simulink model "testbed_simulink_model"  (R2021a)
settings: Solver=FixedStepAuto  StartTime=0.0  StopTime=3  RelTol=1e-3
InitFcn:
  | fsw=10e3;
  | Ts=1/(fsw*50);
  | Vodref=220*sqrt(2);
  | Vdc=700;
  | w0=2*pi*50;
  | 
  | Lf=3.5e-3;
  | Rf=0.1;
  | Cf=50e-6;
  | Lc=0.35e-3;
  | Rc=0.05;
  | 
  | Tci=4/(2*pi*fsw);
  | wci=1/Tci;
  | Kpc=Lf*wci;
  | Kic=Rf*wci;
  | 
  | pm=50;
  | wcv=1/Tci*(1-sind(pm))/(1+sind(pm));
  | wgc=sqrt(wcv*wci);
  | Kpv=Cf*wgc;
  | Kiv=Kpv*wcv;
  | 
  | mp1=5e-5;
  | nq1=3e-3;
  | mp2=5e-5;
  | nq2=3e-3;
  | mp3=5e-5;
  | nq3=3e-3;
libraries: spsabctodq0Lib x15, pid_lib x12, spsThreePhaseSeriesRLCBranchLib x11, spsThreePhaseVIMeasurementLib x6, spsThreePhaseSeriesRLCLoadLib x5, spsThreePhaseBreakerLib x4, spsDCVoltageSourceLib x3, spsGroundLib x3, spsPWMGenerator2LevelLib x3, spsUniversalBridgeLib x3, spsdq0toabcLib x3, spsThreePhaseFaultLib x1
(part 1 of 2)
settings Model: SimulationMode=accelerator  Creator=HP omen  LastModifiedBy=chigo
settings SolverCC: AlgebraicLoopSolver=TrustRegion
settings DataIOCC: ReturnWorkspaceOutputs=off

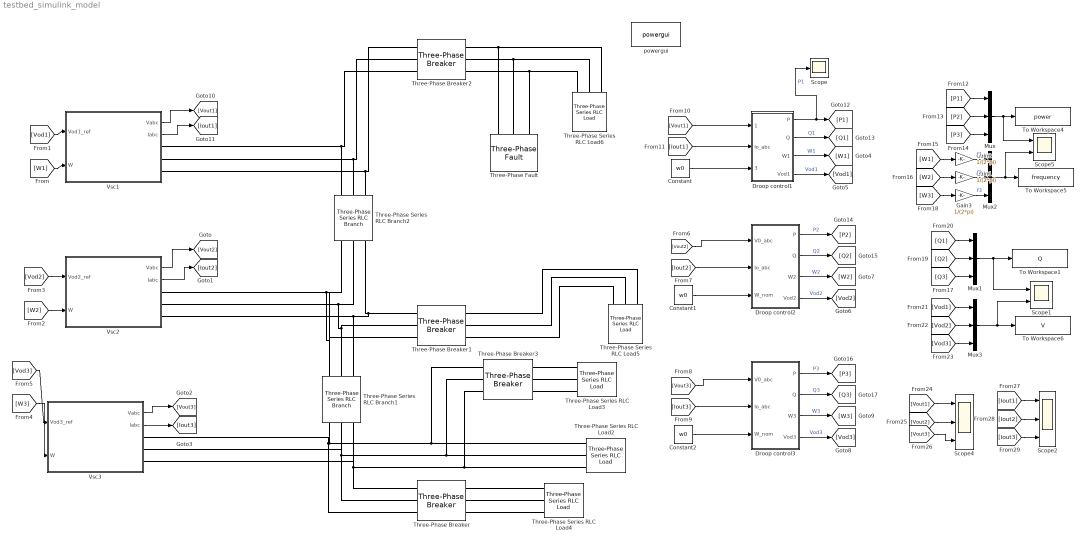
== system testbed_simulink_model ==
  Constant : Constant  Value=w0
  Constant1 : Constant  Value=w0
  Constant2 : Constant  Value=w0
  Droop control1 : Subsystem
  Droop control2 : Subsystem
  Droop control3 : Subsystem
  Gain1 : Gain  Gain=1/(2*pi)
  Gain2 : Gain  Gain=1/(2*pi)
  Gain3 : Gain  Gain=1/(2*pi)
  Mux{,1..3} (4 alike) : Mux  Inputs=3
  Scope : Scope
  Scope1 : Scope  NumInputPorts=2
  Scope2 : Scope  NumInputPorts=3
  Scope4 : Scope  NumInputPorts=3
  Scope5 : Scope  NumInputPorts=2
  Three-Phase Series RLC Branch1 : spsThreePhaseSeriesRLCBranchLib/Three-Phase Series RLC Branch  LConnTagsString=A|B|C  RConnTagsString=A|B|C  BranchType=RL  Resistance=0.15  Inductance=3.5e-4  Capacitance=1e-6  Measurements=Branch voltages
  Three-Phase Series RLC Branch2 : spsThreePhaseSeriesRLCBranchLib/Three-Phase Series RLC Branch  LConnTagsString=A|B|C  RConnTagsString=A|B|C  BranchType=RL  Resistance=0.15  Inductance=3.5e-4  Capacitance=1e-6  Measurements=None
  Three-Phase Series RLC Load2 : spsThreePhaseSeriesRLCLoadLib/Three-Phase Series RLC Load  LConnTagsString=A|B|C  Configuration=Y (grounded)  NominalVoltage=380  Vabc=[1e3 1e3 1e3]  Vabcp=[1e3 1e3 1e3]  NominalFrequency=50  UnbalancedPower=off  ActivePower=6.3e3  InductivePower=1e3  CapacitivePower=0  Pabc=[10e3 9e3 11e3]  QLabc=[100 90 110]  QCabc=[100 90 110]  Pabcp=[10e3 9e3 11e3]  QLabcp=[100 90 110]  QCabcp=[100 90 110]  Measurements=None  LoadType=constant Z
  Three-Phase Series RLC Load3 : spsThreePhaseSeriesRLCLoadLib/Three-Phase Series RLC Load  LConnTagsString=A|B|C  Configuration=Y (grounded)  NominalVoltage=380  Vabc=[1e3 1e3 1e3]  Vabcp=[1e3 1e3 1e3]  NominalFrequency=50  UnbalancedPower=off  ActivePower=2.3e3  InductivePower=0.3e3  CapacitivePower=0  Pabc=[10e3 9e3 11e3]  QLabc=[100 90 110]  QCabc=[100 90 110]  Pabcp=[10e3 9e3 11e3]  QLabcp=[100 90 110]  QCabcp=[100 90 110]  Measurements=None  LoadType=constant Z
  Three-Phase Series RLC Load4 : spsThreePhaseSeriesRLCLoadLib/Three-Phase Series RLC Load  LConnTagsString=A|B|C  Configuration=Y (grounded)  NominalVoltage=380  Vabc=[1e3 1e3 1e3]  Vabcp=[1e3 1e3 1e3]  NominalFrequency=50  UnbalancedPower=off  ActivePower=5.8e3  InductivePower=0.2e3  CapacitivePower=0  Pabc=[10e3 9e3 11e3]  QLabc=[100 90 110]  QCabc=[100 90 110]  Pabcp=[10e3 9e3 11e3]  QLabcp=[100 90 110]  QCabcp=[100 90 110]  Measurements=None  LoadType=constant Z
  Three-Phase Series RLC Load5 : spsThreePhaseSeriesRLCLoadLib/Three-Phase Series RLC Load  LConnTagsString=A|B|C  Configuration=Y (grounded)  NominalVoltage=380  Vabc=[1e3 1e3 1e3]  Vabcp=[1e3 1e3 1e3]  NominalFrequency=50  UnbalancedPower=off  ActivePower=5.8e3  InductivePower=0.2e3  CapacitivePower=0  Pabc=[10e3 9e3 11e3]  QLabc=[100 90 110]  QCabc=[100 90 110]  Pabcp=[10e3 9e3 11e3]  QLabcp=[100 90 110]  QCabcp=[100 90 110]  Measurements=None  LoadType=constant Z
  Three-Phase Series RLC Load6 : spsThreePhaseSeriesRLCLoadLib/Three-Phase Series RLC Load  LConnTagsString=A|B|C  Configuration=Y (grounded)  NominalVoltage=380  Vabc=[1e3 1e3 1e3]  Vabcp=[1e3 1e3 1e3]  NominalFrequency=50  UnbalancedPower=off  ActivePower=5.8e3  InductivePower=0.2e3  CapacitivePower=0  Pabc=[10e3 9e3 11e3]  QLabc=[100 90 110]  QCabc=[100 90 110]  Pabcp=[10e3 9e3 11e3]  QLabcp=[100 90 110]  QCabcp=[100 90 110]  Measurements=None  LoadType=constant Z
  Three-Phase Breaker : spsThreePhaseBreakerLib/Three-Phase Breaker  InitialState=open  SwitchA=on  SwitchB=on  SwitchC=on  SwitchTimes=0  External=off  BreakerResistance=0.01  SnubberResistance=1e6  SnubberCapacitance=inf  Measurements=None
  Three-Phase Breaker1 : spsThreePhaseBreakerLib/Three-Phase Breaker  InitialState=open  SwitchA=on  SwitchB=on  SwitchC=on  SwitchTimes=0  External=off  BreakerResistance=0.01  SnubberResistance=1e6  SnubberCapacitance=inf  Measurements=None
  Three-Phase Breaker2 : spsThreePhaseBreakerLib/Three-Phase Breaker  InitialState=closed  SwitchA=on  SwitchB=on  SwitchC=on  SwitchTimes=0  External=off  BreakerResistance=0.01  SnubberResistance=1e6  SnubberCapacitance=inf  Measurements=None
  Three-Phase Breaker3 : spsThreePhaseBreakerLib/Three-Phase Breaker  InitialState=closed  SwitchA=on  SwitchB=on  SwitchC=on  SwitchTimes=0  External=off  BreakerResistance=0.01  SnubberResistance=1e6  SnubberCapacitance=inf  Measurements=None
  Three-Phase Fault : spsThreePhaseFaultLib/Three-Phase Fault  InitialStates=0  FaultA=off  FaultB=off  FaultC=off  GroundFault=off  SwitchTimes=[2]  External=off  SwitchStatus=NaN  FaultResistance=0.001  GroundResistance=0.01  SnubberResistance=1e6  SnubberCapacitance=inf  Measurements=None
  To Workspace1 : ToWorkspace  VariableName=Q  SaveFormat=Structure With Time  SampleTime=-1
  To Workspace4 : ToWorkspace  VariableName=power  SaveFormat=Structure With Time  SampleTime=-1
  To Workspace5 : ToWorkspace  VariableName=frequency  SaveFormat=Structure With Time  SampleTime=-1
  To Workspace6 : ToWorkspace  VariableName=V  SaveFormat=Structure With Time  SampleTime=-1
  Vsc1 : Subsystem
  Vsc2 : Subsystem
  Vsc3 : Subsystem
  powergui : spspowerguiLib/powergui  Priority=1  SimulationMode=Discrete  SampleTime=Ts  frequency=60  Iterations=50  frequencyindice=0  Pbase=100e6  ErrMax=1e-4  UnitsV=kV  UnitsW=MW  buscounter=0  FunctionMessages=off  echomessages=off  EnableUseOfTLC=off  CurrentSourceSwitches=off  DisableSnubberDevices=off  DisableRonSwitches=off  DisableVfSwitches=off  DisplayEquations=off  AutomaticDiscreteSolvers=off  SolverType=Tustin/Backward Euler (TBE)  Interpol=off  ExternalGateDelay=off  methode=off  Ts=100  x0status=blocks  SPID=on  SwTol=0  HookPort=off  NonlinearTolerance=1e-4  nMaxIteration=100  ContinueOnMaxIteration=off  RestoreLinks=warning  ResistiveCurrentMeasurement=off  Frange=[0:2:500]  Ylog=off  Xlog=on  ShowGrid=off  save=off  variable=ZData  structure=0  ZoomFFT=off  StartTime=0.0  cycles=1  DisplayStyle=1  fundamental=60  FreqAxis=off  MaxFrequency=1000  frequencyindicesteady=1  RmsSteady=1  display=off
  wires:
  Vsc2/1(Vabc) -> [Vout2]
  Vsc3/1(Vabc) -> [Vout3]
  Vsc2/2(Iabc) -> [Iout2]
  Vsc3/2(Iabc) -> [Iout3]
  Constant/1 -> Droop control1/3(W_nom)
  Droop control1/3(W1) -> [W1]  "W1"
  Droop control1/4(Vod1) -> [Vod1]  "Vod1"
  [Vod1] -> Vsc1/1(Vod1_ref)
  [W1] -> Vsc1/2(W)
  [W3] -> Vsc3/2(W)
  [Vod3] -> Vsc3/1(Vod3_ref)
  [W2] -> Vsc2/2(W)
  [Vod2] -> Vsc2/1(Vod2_ref)
  [Vout3] -> Droop control3/1(V0_abc)
  [Iout3] -> Droop control3/2(Io_abc)
  [Vout2] -> Droop control2/1(V0_abc)
  [Iout2] -> Droop control2/2(Io_abc)
  Constant1/1 -> Droop control2/3(W_nom)
  Constant2/1 -> Droop control3/3(W_nom)
  Droop control2/3(W2) -> [W2]  "W2"
  Droop control2/4(Vod2) -> [Vod2]  "Vod2"
  Droop control3/4(Vod3) -> [Vod3]  "Vod3"
  Droop control3/3(W3) -> [W3]  "W3"
  Vsc1/1(Vabc) -> [Vout1]
  Vsc1/2(Iabc) -> [Iout1]
  [Iout1] -> Droop control1/2(Io_abc)
  [Vout1] -> Droop control1/1(V0_abc)
  Droop control1/1(P) -> Scope/1, [P1]  "P1"
  Droop control1/2(Q) -> [Q1]  "Q1"
  Droop control2/1(P) -> [P2]  "P2"
  Droop control2/2(Q) -> [Q2]  "Q2"
  Droop control3/1(P) -> [P3]  "P3"
  Droop control3/2(Q) -> [Q3]  "Q3"
  [W1] -> Gain2/1
  [W2] -> Gain1/1
  [W3] -> Gain3/1
  [P2] -> Mux/2
  [P1] -> Mux/1
  [P3] -> Mux/3
  [Q1] -> Mux1/1
  [Q2] -> Mux1/2
  [Q3] -> Mux1/3
  Gain2/1 -> Mux2/1  "f1"
  Gain1/1 -> Mux2/2  "f2"
  Gain3/1 -> Mux2/3  "f3"
  [Vod1] -> Mux3/1
  [Vod2] -> Mux3/2
  [Vod3] -> Mux3/3
  Mux1/1 -> To Workspace1/1, Scope1/1
  Mux3/1 -> To Workspace6/1, Scope1/2
  Mux/1 -> Scope5/1, To Workspace4/1
  Mux2/1 -> To Workspace5/1, Scope5/2
  [Vout1] -> Scope4/1
  [Vout2] -> Scope4/2
  [Vout3] -> Scope4/3
  [Iout1] -> Scope2/1
  [Iout2] -> Scope2/2
  [Iout3] -> Scope2/3
  connections:
  Three-Phase Breaker2/LConn1 -- Vsc1/RConn1 -- Three-Phase Series RLC Branch2/LConn1
  Three-Phase Series RLC Load2/LConn1 -- Three-Phase Breaker3/LConn1 -- Vsc3/RConn1 -- Three-Phase Breaker/LConn1 -- Three-Phase Series RLC Branch1/RConn1
  Three-Phase Series RLC Branch2/LConn2 -- Three-Phase Breaker2/LConn2 -- Vsc1/RConn2
  Three-Phase Series RLC Branch2/LConn3 -- Three-Phase Breaker2/LConn3 -- Vsc1/RConn3
  Three-Phase Series RLC Load2/LConn2 -- Three-Phase Breaker3/LConn2 -- Three-Phase Series RLC Branch1/RConn2 -- Vsc3/RConn2 -- Three-Phase Breaker/LConn2
  Three-Phase Breaker/RConn3 -- Three-Phase Series RLC Load4/LConn1
  Three-Phase Breaker/RConn2 -- Three-Phase Series RLC Load4/LConn2
  Three-Phase Breaker/RConn1 -- Three-Phase Series RLC Load4/LConn3
  Three-Phase Series RLC Load5/LConn1 -- Three-Phase Breaker1/RConn1
  Three-Phase Series RLC Load5/LConn2 -- Three-Phase Breaker1/RConn2
  Three-Phase Series RLC Load5/LConn3 -- Three-Phase Breaker1/RConn3
  Three-Phase Series RLC Load6/LConn1 -- Three-Phase Fault/LConn1 -- Three-Phase Breaker2/RConn1
  Three-Phase Series RLC Load6/LConn2 -- Three-Phase Breaker2/RConn2 -- Three-Phase Fault/LConn2
  Three-Phase Series RLC Load6/LConn3 -- Three-Phase Fault/LConn3 -- Three-Phase Breaker2/RConn3
  Three-Phase Series RLC Branch2/RConn3 -- Three-Phase Breaker1/LConn3 -- Vsc2/RConn3 -- Three-Phase Series RLC Branch1/LConn3
  Three-Phase Series RLC Branch2/RConn1 -- Vsc2/RConn1 -- Three-Phase Breaker1/LConn1 -- Three-Phase Series RLC Branch1/LConn1
  Three-Phase Series RLC Branch1/LConn2 -- Three-Phase Breaker1/LConn2 -- Vsc2/RConn2 -- Three-Phase Series RLC Branch2/RConn2
  Three-Phase Series RLC Load2/LConn3 -- Three-Phase Breaker3/LConn3 -- Three-Phase Series RLC Branch1/RConn3 -- Vsc3/RConn3 -- Three-Phase Breaker/LConn3
  Three-Phase Breaker3/RConn1 -- Three-Phase Series RLC Load3/LConn1
  Three-Phase Breaker3/RConn2 -- Three-Phase Series RLC Load3/LConn2
  Three-Phase Breaker3/RConn3 -- Three-Phase Series RLC Load3/LConn3

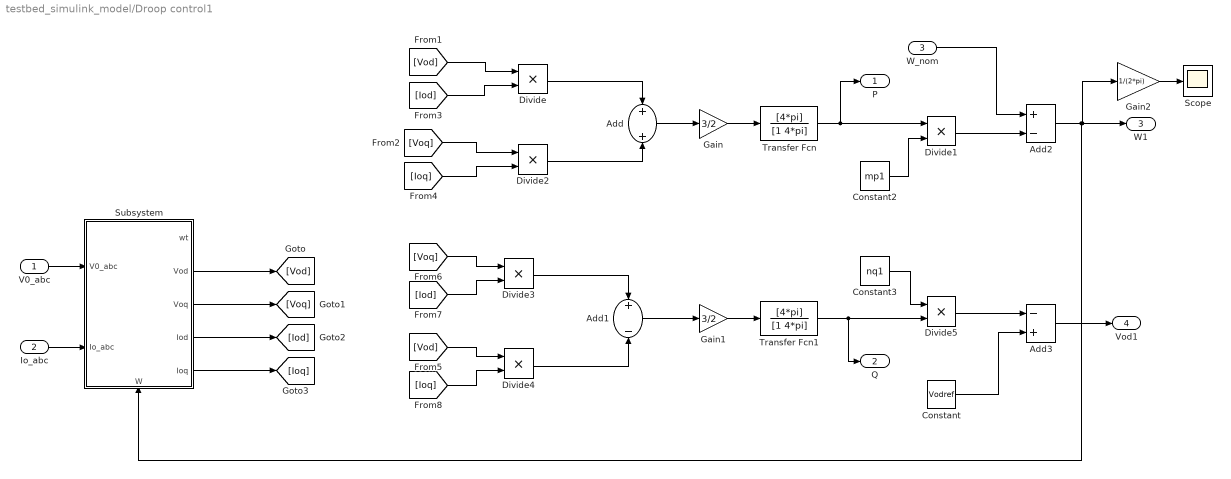
== system testbed_simulink_model/Droop control1 ==
  V0_abc : Inport
  Io_abc : Inport  Port=2
  W_nom : Inport  Port=3
  Add : Sum
  Add1 : Sum  Inputs=+-
  Add2 : Sum  Inputs=+-
  Add3 : Sum  Inputs=-+
  Constant : Constant  Value=Vodref
  Constant2 : Constant  Value=mp1
  Constant3 : Constant  Value=nq1
  Divide{,1..5} (6 alike) : Product  Inputs=**
  Gain : Gain  Gain=3/2
  Gain1 : Gain  Gain=3/2
  Gain2 : Gain  Gain=1/(2*pi)
  Scope : Scope
  Subsystem : Subsystem
      settings: PortSchema="{\"entries\":[{\"content\":{\"sides\":[{\"content\":{\"connectorIds\":[\"In1\",\"In2\"]},\"type\":\"ConnectorPlacement.EquallySpacedRectSide\",\"uuid\":\"3c0ce44c-1409-4df9-aab1-2e1a82b43481\"},{\"content\":{\"connectorIds\":[\"Out1\",\"Out2\",\"Out3\",\"Out4\",\"Out5\"],\"side\":\"RIGHT\"},\"type\":\"ConnectorPlacement.EquallySpacedRectSide\",\"uuid\":\"4a9336a4-679f-4f93-987c-a9f8549bd21c\"},{\"content\":{\"connectorIds\":[],\"side\":\"TOP\"},\"type\":\"ConnectorPlacement.EquallySpacedRectSide\",\"uuid\":\"6340f487-ff74-466e-845e-7d1050881641\"},{\"content\":{\"connectorIds\":[\"In3\"],\"side\":\"BOTTOM\"},\"type\":\"ConnectorPlacement.EquallySpacedRectSide\",\"uuid\":\"1e1d92d0-8955-434a-9fbd-76af504505ea\"}]},\"type\":\"ConnectorPlacement.EquallySpacedConnector\",\"uuid\":\"bfddd833-a64a-4f18-a4bd-88042aac52a3\"}],\"packageUris\":[\"http://schema.mathworks.com/mf0/Connector/R2020b\"],\"version\":\"1.0\"}"
  Transfer Fcn : TransferFcn  Numerator=[4*pi]  Denominator=[1 4*pi]
  Transfer Fcn1 : TransferFcn  Numerator=[4*pi]  Denominator=[1 4*pi]
  P : Outport
  Q : Outport  Port=2
  W1 : Outport  Port=3
  Vod1 : Outport  Port=4
  wires:
  Subsystem/2(Vod) -> [Vod]
  Subsystem/3(Voq) -> [Voq]
  Subsystem/4(Iod) -> [Iod]
  Subsystem/5(Ioq) -> [Ioq]
  [Vod] -> Divide/1
  [Iod] -> Divide/2
  [Voq] -> Divide2/1
  [Ioq] -> Divide2/2
  Divide/1 -> Add/1
  Divide2/1 -> Add/2
  Add/1 -> Gain/1
  [Voq] -> Divide3/1
  [Iod] -> Divide3/2
  [Vod] -> Divide4/1
  [Ioq] -> Divide4/2
  Divide3/1 -> Add1/1
  Divide4/1 -> Add1/2
  Add1/1 -> Gain1/1
  W_nom/1 -> Add2/1
  Divide1/1 -> Add2/2
  Divide5/1 -> Add3/1
  Constant/1 -> Add3/2
  Constant2/1 -> Divide1/2
  Constant3/1 -> Divide5/1
  Add2/1 -> Gain2/1, W1/1, Subsystem/3(W)
  Add3/1 -> Vod1/1
  Gain/1 -> Transfer Fcn/1
  Transfer Fcn/1 -> P/1, Divide1/1
  Gain1/1 -> Transfer Fcn1/1
  Transfer Fcn1/1 -> Q/1, Divide5/2
  Io_abc/1 -> Subsystem/2(Io_abc)
  V0_abc/1 -> Subsystem/1(V0_abc)
  Gain2/1 -> Scope/1

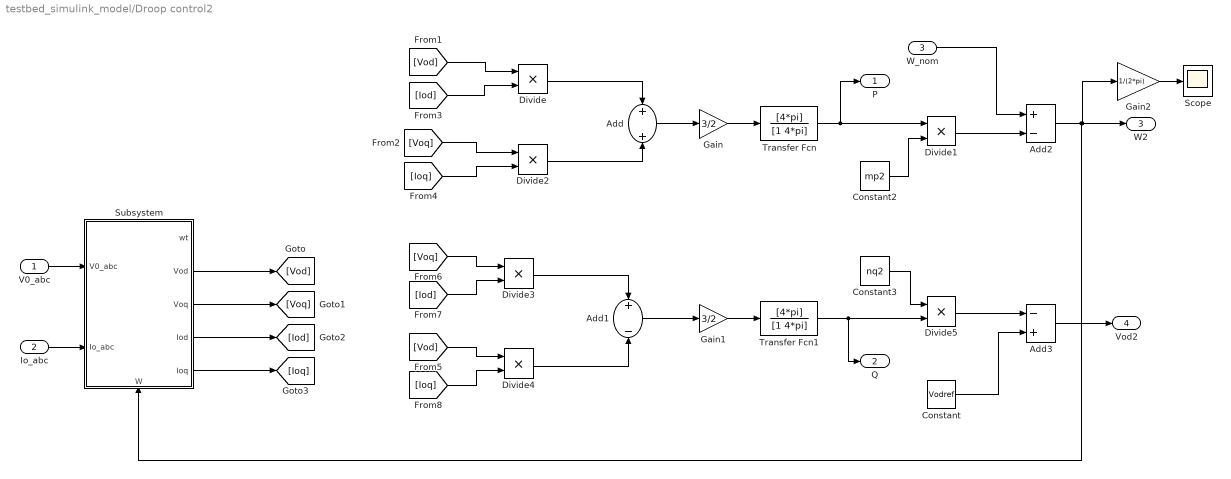
== system testbed_simulink_model/Droop control2 ==
  V0_abc : Inport
  Io_abc : Inport  Port=2
  W_nom : Inport  Port=3
  Add : Sum
  Add1 : Sum  Inputs=+-
  Add2 : Sum  Inputs=+-
  Add3 : Sum  Inputs=-+
  Constant : Constant  Value=Vodref
  Constant2 : Constant  Value=mp2
  Constant3 : Constant  Value=nq2
  Divide{,1..5} (6 alike) : Product  Inputs=**
  Gain : Gain  Gain=3/2
  Gain1 : Gain  Gain=3/2
  Gain2 : Gain  Gain=1/(2*pi)
  Scope : Scope
  Subsystem : Subsystem
      settings: PortSchema="{\"entries\":[{\"content\":{\"sides\":[{\"content\":{\"connectorIds\":[\"In1\",\"In2\"]},\"type\":\"ConnectorPlacement.EquallySpacedRectSide\",\"uuid\":\"3c0ce44c-1409-4df9-aab1-2e1a82b43481\"},{\"content\":{\"connectorIds\":[\"Out1\",\"Out2\",\"Out3\",\"Out4\",\"Out5\"],\"side\":\"RIGHT\"},\"type\":\"ConnectorPlacement.EquallySpacedRectSide\",\"uuid\":\"4a9336a4-679f-4f93-987c-a9f8549bd21c\"},{\"content\":{\"connectorIds\":[],\"side\":\"TOP\"},\"type\":\"ConnectorPlacement.EquallySpacedRectSide\",\"uuid\":\"6340f487-ff74-466e-845e-7d1050881641\"},{\"content\":{\"connectorIds\":[\"In3\"],\"side\":\"BOTTOM\"},\"type\":\"ConnectorPlacement.EquallySpacedRectSide\",\"uuid\":\"1e1d92d0-8955-434a-9fbd-76af504505ea\"}]},\"type\":\"ConnectorPlacement.EquallySpacedConnector\",\"uuid\":\"bfddd833-a64a-4f18-a4bd-88042aac52a3\"}],\"packageUris\":[\"http://schema.mathworks.com/mf0/Connector/R2020b\"],\"version\":\"1.0\"}"
  Transfer Fcn : TransferFcn  Numerator=[4*pi]  Denominator=[1 4*pi]
  Transfer Fcn1 : TransferFcn  Numerator=[4*pi]  Denominator=[1 4*pi]
  P : Outport
  Q : Outport  Port=2
  W2 : Outport  Port=3
  Vod2 : Outport  Port=4
  wires:
  Subsystem/2(Vod) -> [Vod]
  Subsystem/3(Voq) -> [Voq]
  Subsystem/4(Iod) -> [Iod]
  Subsystem/5(Ioq) -> [Ioq]
  [Vod] -> Divide/1
  [Iod] -> Divide/2
  [Voq] -> Divide2/1
  [Ioq] -> Divide2/2
  Divide/1 -> Add/1
  Divide2/1 -> Add/2
  Add/1 -> Gain/1
  [Voq] -> Divide3/1
  [Iod] -> Divide3/2
  [Vod] -> Divide4/1
  [Ioq] -> Divide4/2
  Divide3/1 -> Add1/1
  Divide4/1 -> Add1/2
  Add1/1 -> Gain1/1
  W_nom/1 -> Add2/1
  Divide1/1 -> Add2/2
  Divide5/1 -> Add3/1
  Constant/1 -> Add3/2
  Constant2/1 -> Divide1/2
  Constant3/1 -> Divide5/1
  Add2/1 -> Gain2/1, W2/1, Subsystem/3(W)
  Add3/1 -> Vod2/1
  Gain/1 -> Transfer Fcn/1
  Transfer Fcn/1 -> P/1, Divide1/1
  Gain1/1 -> Transfer Fcn1/1
  Transfer Fcn1/1 -> Q/1, Divide5/2
  Io_abc/1 -> Subsystem/2(Io_abc)
  V0_abc/1 -> Subsystem/1(V0_abc)
  Gain2/1 -> Scope/1

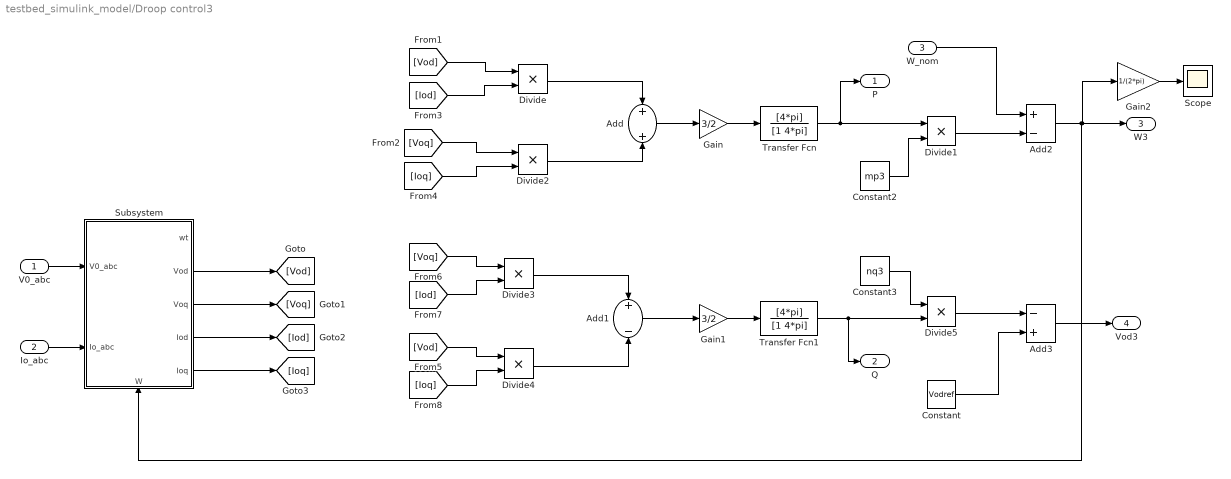
== system testbed_simulink_model/Droop control3 ==
  V0_abc : Inport
  Io_abc : Inport  Port=2
  W_nom : Inport  Port=3
  Add : Sum
  Add1 : Sum  Inputs=+-
  Add2 : Sum  Inputs=+-
  Add3 : Sum  Inputs=-+
  Constant : Constant  Value=Vodref
  Constant2 : Constant  Value=mp3
  Constant3 : Constant  Value=nq3
  Divide{,1..5} (6 alike) : Product  Inputs=**
  Gain : Gain  Gain=3/2
  Gain1 : Gain  Gain=3/2
  Gain2 : Gain  Gain=1/(2*pi)
  Scope : Scope
  Subsystem : Subsystem
      settings: PortSchema="{\"entries\":[{\"content\":{\"sides\":[{\"content\":{\"connectorIds\":[\"In1\",\"In2\"]},\"type\":\"ConnectorPlacement.EquallySpacedRectSide\",\"uuid\":\"3c0ce44c-1409-4df9-aab1-2e1a82b43481\"},{\"content\":{\"connectorIds\":[\"Out1\",\"Out2\",\"Out3\",\"Out4\",\"Out5\"],\"side\":\"RIGHT\"},\"type\":\"ConnectorPlacement.EquallySpacedRectSide\",\"uuid\":\"4a9336a4-679f-4f93-987c-a9f8549bd21c\"},{\"content\":{\"connectorIds\":[],\"side\":\"TOP\"},\"type\":\"ConnectorPlacement.EquallySpacedRectSide\",\"uuid\":\"6340f487-ff74-466e-845e-7d1050881641\"},{\"content\":{\"connectorIds\":[\"In3\"],\"side\":\"BOTTOM\"},\"type\":\"ConnectorPlacement.EquallySpacedRectSide\",\"uuid\":\"1e1d92d0-8955-434a-9fbd-76af504505ea\"}]},\"type\":\"ConnectorPlacement.EquallySpacedConnector\",\"uuid\":\"bfddd833-a64a-4f18-a4bd-88042aac52a3\"}],\"packageUris\":[\"http://schema.mathworks.com/mf0/Connector/R2020b\"],\"version\":\"1.0\"}"
  Transfer Fcn : TransferFcn  Numerator=[4*pi]  Denominator=[1 4*pi]
  Transfer Fcn1 : TransferFcn  Numerator=[4*pi]  Denominator=[1 4*pi]
  P : Outport
  Q : Outport  Port=2
  W3 : Outport  Port=3
  Vod3 : Outport  Port=4
  wires:
  Subsystem/2(Vod) -> [Vod]
  Subsystem/3(Voq) -> [Voq]
  Subsystem/4(Iod) -> [Iod]
  Subsystem/5(Ioq) -> [Ioq]
  [Vod] -> Divide/1
  [Iod] -> Divide/2
  [Voq] -> Divide2/1
  [Ioq] -> Divide2/2
  Divide/1 -> Add/1
  Divide2/1 -> Add/2
  Add/1 -> Gain/1
  [Voq] -> Divide3/1
  [Iod] -> Divide3/2
  [Vod] -> Divide4/1
  [Ioq] -> Divide4/2
  Divide3/1 -> Add1/1
  Divide4/1 -> Add1/2
  Add1/1 -> Gain1/1
  W_nom/1 -> Add2/1
  Divide1/1 -> Add2/2
  Divide5/1 -> Add3/1
  Constant/1 -> Add3/2
  Constant2/1 -> Divide1/2
  Constant3/1 -> Divide5/1
  Add2/1 -> Gain2/1, W3/1, Subsystem/3(W)
  Add3/1 -> Vod3/1
  Gain/1 -> Transfer Fcn/1
  Transfer Fcn/1 -> P/1, Divide1/1
  Gain1/1 -> Transfer Fcn1/1
  Transfer Fcn1/1 -> Q/1, Divide5/2
  Io_abc/1 -> Subsystem/2(Io_abc)
  V0_abc/1 -> Subsystem/1(V0_abc)
  Gain2/1 -> Scope/1

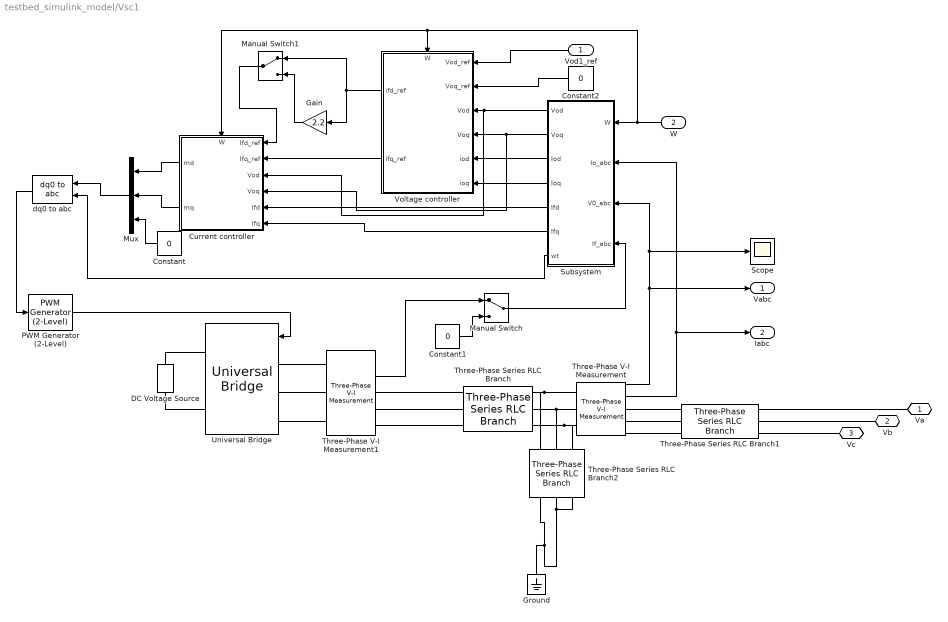
== system testbed_simulink_model/Vsc1 ==
  Vod1_ref : Inport
  W : Inport  Port=2
  Constant : Constant  Value=0
  Constant1 : Constant  Value=0
  Constant2 : Constant  Value=0
  Current controller : Subsystem
      settings: PortSchema="{\"entries\":[{\"content\":{\"sides\":[{\"content\":{\"connectorIds\":[\"In1\",\"In2\",\"In3\",\"In4\",\"In5\",\"In6\"]},\"type\":\"ConnectorPlacement.EquallySpacedRectSide\",\"uuid\":\"afbd0cd8-be12-4bd7-a6dd-f7dac5cf4512\"},{\"content\":{\"connectorIds\":[\"Out1\",\"Out2\"],\"side\":\"RIGHT\"},\"type\":\"ConnectorPlacement.EquallySpacedRectSide\",\"uuid\":\"a2288591-3041-41c1-b291-e9e060e5938f\"},{\"content\":{\"connectorIds\":[\"In7\"],\"side\":\"TOP\"},\"type\":\"ConnectorPlacement.EquallySpacedRectSide\",\"uuid\":\"6bd258a4-7022-4004-b2e3-8400b1f87dc6\"}]},\"type\":\"ConnectorPlacement.EquallySpacedConnector\",\"uuid\":\"ef76f81b-f821-49f2-9550-8127a934c8c3\"}],\"packageUris\":[\"http://schema.mathworks.com/mf0/Connector/R2020b\"],\"version\":\"1.0\"}"
  DC Voltage Source : spsDCVoltageSourceLib/DC Voltage Source  Amplitude=Vdc  Measurements=None
  Gain : Gain  Gain=2.2
  Ground : spsGroundLib/Ground  LConnTagsString=a
  Manual Switch : ManualSwitch
  Manual Switch1 : ManualSwitch
  Mux : Mux  Inputs=3
  PWM Generator (2-Level) : spsPWMGenerator2LevelLib/PWM Generator (2-Level)  ModulatorType=Three-phase bridge (6 pulses)  ModulatorMode=Unsynchronized  Fc=fsw  Pc=0  nF=27  MinMax="[ -1  1 ]"  SamplingTechnique=Natural  ModulatingSignals=off  m=0.8  Freq=60  Phase=0  Ts=0  ShowCarrierOutport=off
  Scope : Scope
  Subsystem : Subsystem
  Three-Phase Series RLC Branch : spsThreePhaseSeriesRLCBranchLib/Three-Phase Series RLC Branch  LConnTagsString=A|B|C  RConnTagsString=A|B|C  BranchType=RL  Resistance=Rf  Inductance=Lf  Capacitance=1e-6  Measurements=None
  Three-Phase Series RLC Branch1 : spsThreePhaseSeriesRLCBranchLib/Three-Phase Series RLC Branch  LConnTagsString=A|B|C  RConnTagsString=A|B|C  BranchType=RL  Resistance=Rc  Inductance=Lc  Capacitance=1e-6  Measurements=None
  Three-Phase Series RLC Branch2 : spsThreePhaseSeriesRLCBranchLib/Three-Phase Series RLC Branch  LConnTagsString=A|B|C  RConnTagsString=A|B|C  BranchType=C  Resistance=1  Inductance=1e-3  Capacitance=Cf  Measurements=None
  Three-Phase V-I Measurement : spsThreePhaseVIMeasurementLib/Three-Phase V-I Measurement  VoltageMeasurement=phase-to-ground  SetLabelV=off  LabelV=Vabc  Vpu=off  VpuLL=off  CurrentMeasurement=yes  SetLabelI=off  LabelI=Iabc  Ipu=off  Pbase=100e6  Vbase=500e3  OutputType=Complex  PhasorSimulation=off  PSBequivalent=0
  Three-Phase V-I Measurement1 : spsThreePhaseVIMeasurementLib/Three-Phase V-I Measurement  VoltageMeasurement=phase-to-ground  SetLabelV=off  LabelV=Vabc  Vpu=off  VpuLL=off  CurrentMeasurement=yes  SetLabelI=off  LabelI=Iabc  Ipu=off  Pbase=100e6  Vbase=500e3  OutputType=Complex  PhasorSimulation=off  PSBequivalent=0
  Universal Bridge : spsUniversalBridgeLib/Universal Bridge  Arms=3  SnubberResistance=1e5  SnubberCapacitance=inf  Device=IGBT / Diodes  Ron=1e-3  Lon=0  ForwardVoltages="[  0  0  ]"  ForwardVoltage=0  GTOparameters=[ 10e-6 , 20e-6 ]  IGBTparameters=[ 1e-6 , 2e-6 ]  Measurements=None  Measurements_2=None  converterType=Rectifier
  Voltage controller : Subsystem
      settings: PortSchema="{\"entries\":[{\"content\":{\"sides\":[{\"content\":{\"connectorIds\":[\"In1\",\"In2\",\"In3\",\"In4\",\"In5\",\"In6\"]},\"type\":\"ConnectorPlacement.EquallySpacedRectSide\",\"uuid\":\"afbd0cd8-be12-4bd7-a6dd-f7dac5cf4512\"},{\"content\":{\"connectorIds\":[\"Out1\",\"Out2\"],\"side\":\"RIGHT\"},\"type\":\"ConnectorPlacement.EquallySpacedRectSide\",\"uuid\":\"a2288591-3041-41c1-b291-e9e060e5938f\"},{\"content\":{\"connectorIds\":[\"In7\"],\"side\":\"TOP\"},\"type\":\"ConnectorPlacement.EquallySpacedRectSide\",\"uuid\":\"6bd258a4-7022-4004-b2e3-8400b1f87dc6\"}]},\"type\":\"ConnectorPlacement.EquallySpacedConnector\",\"uuid\":\"ef76f81b-f821-49f2-9550-8127a934c8c3\"}],\"packageUris\":[\"http://schema.mathworks.com/mf0/Connector/R2020b\"],\"version\":\"1.0\"}"
  dq0 to abc : spsdq0toabcLib/dq0 to abc  Alignment=90 degrees behind phase A axis
  Va : PMIOPort  Side=Right
  Vb : PMIOPort  Port=2  Side=Right
  Vc : PMIOPort  Port=3  Side=Right
  Vabc : Outport
  Iabc : Outport  Port=2
  wires:
  Constant2/1 -> Voltage controller/2(Voq_ref)
  dq0 to abc/1 -> PWM Generator (2-Level)/1
  Subsystem/5(Ifd) -> Current controller/5(Ifd)
  Subsystem/2(Voq) -> Current controller/4(Voq), Voltage controller/4(Voq)
  Vod1_ref/1 -> Voltage controller/1(Vod_ref)
  Subsystem/6(Ifq) -> Current controller/6(Ifq)
  Subsystem/3(Iod) -> Voltage controller/5(iod)
  Voltage controller/2(ifq_ref) -> Current controller/2(Ifq_ref)
  Subsystem/4(Ioq) -> Voltage controller/6(ioq)
  Three-Phase V-I Measurement/2 -> Iabc/1, Subsystem/2(Io_abc)
  PWM Generator (2-Level)/1 -> Universal Bridge/1
  Constant/1 -> Mux/3
  Current controller/2(mq) -> Mux/2
  Current controller/1(md) -> Mux/1
  Subsystem/1(Vod) -> Current controller/3(Vod), Voltage controller/3(Vod)
  Subsystem/7(wt) -> dq0 to abc/2
  Mux/1 -> dq0 to abc/1
  Three-Phase V-I Measurement/1 -> Vabc/1, Scope/1, Subsystem/3(V0_abc)
  W/1 -> Subsystem/1(W), Current controller/7(W), Voltage controller/7(W)
  Voltage controller/1(ifd_ref) -> Gain/1, Manual Switch1/1
  Constant1/1 -> Manual Switch/2
  Manual Switch/1 -> Subsystem/4(If_abc)
  Three-Phase V-I Measurement1/2 -> Manual Switch/1
  Gain/1 -> Manual Switch1/2
  Manual Switch1/1 -> Current controller/1(Ifd_ref)
  connections:
  DC Voltage Source/LConn1 -- Universal Bridge/RConn2
  Three-Phase Series RLC Branch/LConn1 -- Three-Phase V-I Measurement1/RConn1
  Three-Phase V-I Measurement/LConn1 -- Three-Phase Series RLC Branch2/LConn1 -- Three-Phase Series RLC Branch/RConn1
  Three-Phase V-I Measurement1/LConn1 -- Universal Bridge/LConn1
  Three-Phase Series RLC Branch/LConn2 -- Three-Phase V-I Measurement1/RConn2
  Three-Phase V-I Measurement/RConn1 -- Three-Phase Series RLC Branch1/LConn1
  Three-Phase V-I Measurement/RConn2 -- Three-Phase Series RLC Branch1/LConn2
  Three-Phase Series RLC Branch2/RConn1 -- Three-Phase Series RLC Branch2/RConn2 -- Three-Phase Series RLC Branch2/RConn3 -- Ground/LConn1
  DC Voltage Source/RConn1 -- Universal Bridge/RConn1
  Three-Phase V-I Measurement/LConn2 -- Three-Phase Series RLC Branch/RConn2 -- Three-Phase Series RLC Branch2/LConn2
  Three-Phase V-I Measurement/LConn3 -- Three-Phase Series RLC Branch/RConn3 -- Three-Phase Series RLC Branch2/LConn3
  Three-Phase V-I Measurement1/LConn2 -- Universal Bridge/LConn2
  Three-Phase V-I Measurement1/LConn3 -- Universal Bridge/LConn3
  Three-Phase V-I Measurement/RConn3 -- Three-Phase Series RLC Branch1/LConn3
  Vb/RConn1 -- Three-Phase Series RLC Branch1/RConn2
  Three-Phase Series RLC Branch1/RConn3 -- Vc/RConn1
  Three-Phase Series RLC Branch1/RConn1 -- Va/RConn1
  Three-Phase V-I Measurement1/RConn3 -- Three-Phase Series RLC Branch/LConn3

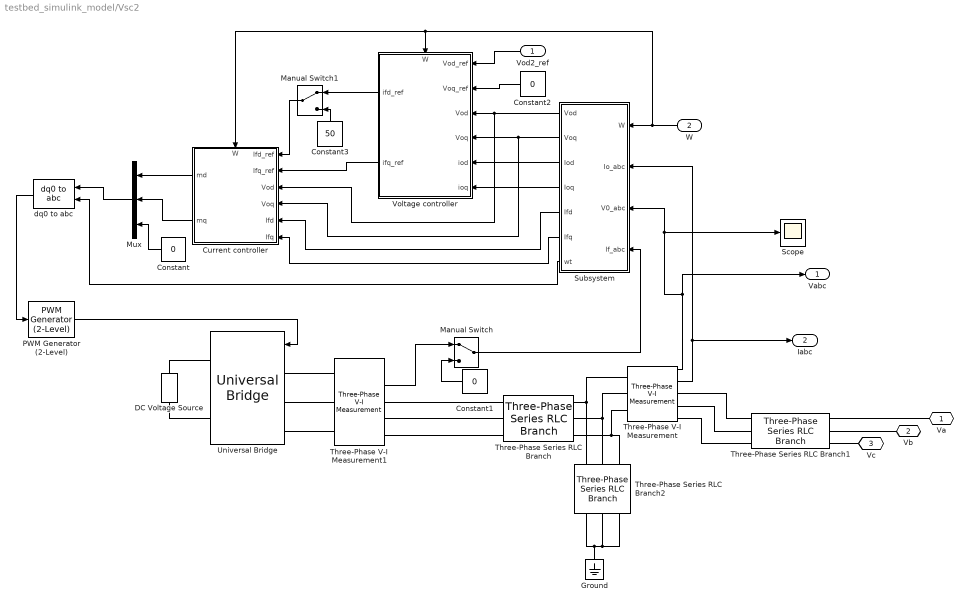
== system testbed_simulink_model/Vsc2 ==
  Vod2_ref : Inport
  W : Inport  Port=2
  Constant : Constant  Value=0
  Constant1 : Constant  Value=0
  Constant2 : Constant  Value=0
  Constant3 : Constant  Value=50
  Current controller : Subsystem
      settings: PortSchema="{\"entries\":[{\"content\":{\"sides\":[{\"content\":{\"connectorIds\":[\"In1\",\"In2\",\"In3\",\"In4\",\"In5\",\"In6\"]},\"type\":\"ConnectorPlacement.EquallySpacedRectSide\",\"uuid\":\"afbd0cd8-be12-4bd7-a6dd-f7dac5cf4512\"},{\"content\":{\"connectorIds\":[\"Out1\",\"Out2\"],\"side\":\"RIGHT\"},\"type\":\"ConnectorPlacement.EquallySpacedRectSide\",\"uuid\":\"a2288591-3041-41c1-b291-e9e060e5938f\"},{\"content\":{\"connectorIds\":[\"In7\"],\"side\":\"TOP\"},\"type\":\"ConnectorPlacement.EquallySpacedRectSide\",\"uuid\":\"6bd258a4-7022-4004-b2e3-8400b1f87dc6\"}]},\"type\":\"ConnectorPlacement.EquallySpacedConnector\",\"uuid\":\"ef76f81b-f821-49f2-9550-8127a934c8c3\"}],\"packageUris\":[\"http://schema.mathworks.com/mf0/Connector/R2020b\"],\"version\":\"1.0\"}"
  DC Voltage Source : spsDCVoltageSourceLib/DC Voltage Source  Amplitude=Vdc  Measurements=None
  Ground : spsGroundLib/Ground  LConnTagsString=a
  Manual Switch : ManualSwitch
  Manual Switch1 : ManualSwitch
  Mux : Mux  Inputs=3
  PWM Generator (2-Level) : spsPWMGenerator2LevelLib/PWM Generator (2-Level)  ModulatorType=Three-phase bridge (6 pulses)  ModulatorMode=Unsynchronized  Fc=fsw  Pc=0  nF=27  MinMax="[ -1  1 ]"  SamplingTechnique=Natural  ModulatingSignals=off  m=0.8  Freq=60  Phase=0  Ts=0  ShowCarrierOutport=off
  Scope : Scope
  Subsystem : Subsystem
  Three-Phase Series RLC Branch : spsThreePhaseSeriesRLCBranchLib/Three-Phase Series RLC Branch  LConnTagsString=A|B|C  RConnTagsString=A|B|C  BranchType=RL  Resistance=Rf  Inductance=Lf  Capacitance=1e-6  Measurements=None
  Three-Phase Series RLC Branch1 : spsThreePhaseSeriesRLCBranchLib/Three-Phase Series RLC Branch  LConnTagsString=A|B|C  RConnTagsString=A|B|C  BranchType=RL  Resistance=Rc  Inductance=Lc  Capacitance=1e-6  Measurements=None
  Three-Phase Series RLC Branch2 : spsThreePhaseSeriesRLCBranchLib/Three-Phase Series RLC Branch  LConnTagsString=A|B|C  RConnTagsString=A|B|C  BranchType=C  Resistance=1  Inductance=1e-3  Capacitance=Cf  Measurements=None
  Three-Phase V-I Measurement : spsThreePhaseVIMeasurementLib/Three-Phase V-I Measurement  VoltageMeasurement=phase-to-ground  SetLabelV=off  LabelV=Vabc  Vpu=off  VpuLL=off  CurrentMeasurement=yes  SetLabelI=off  LabelI=Iabc  Ipu=off  Pbase=100e6  Vbase=500e3  OutputType=Complex  PhasorSimulation=off  PSBequivalent=0
  Three-Phase V-I Measurement1 : spsThreePhaseVIMeasurementLib/Three-Phase V-I Measurement  VoltageMeasurement=phase-to-ground  SetLabelV=off  LabelV=Vabc  Vpu=off  VpuLL=off  CurrentMeasurement=yes  SetLabelI=off  LabelI=Iabc  Ipu=off  Pbase=100e6  Vbase=500e3  OutputType=Complex  PhasorSimulation=off  PSBequivalent=0
  Universal Bridge : spsUniversalBridgeLib/Universal Bridge  Arms=3  SnubberResistance=1e5  SnubberCapacitance=inf  Device=IGBT / Diodes  Ron=1e-3  Lon=0  ForwardVoltages="[  0  0  ]"  ForwardVoltage=0  GTOparameters=[ 10e-6 , 20e-6 ]  IGBTparameters=[ 1e-6 , 2e-6 ]  Measurements=None  Measurements_2=None  converterType=Rectifier
  Voltage controller : Subsystem
      settings: PortSchema="{\"entries\":[{\"content\":{\"sides\":[{\"content\":{\"connectorIds\":[\"In1\",\"In2\",\"In3\",\"In4\",\"In5\",\"In6\"]},\"type\":\"ConnectorPlacement.EquallySpacedRectSide\",\"uuid\":\"afbd0cd8-be12-4bd7-a6dd-f7dac5cf4512\"},{\"content\":{\"connectorIds\":[\"Out1\",\"Out2\"],\"side\":\"RIGHT\"},\"type\":\"ConnectorPlacement.EquallySpacedRectSide\",\"uuid\":\"a2288591-3041-41c1-b291-e9e060e5938f\"},{\"content\":{\"connectorIds\":[\"In7\"],\"side\":\"TOP\"},\"type\":\"ConnectorPlacement.EquallySpacedRectSide\",\"uuid\":\"6bd258a4-7022-4004-b2e3-8400b1f87dc6\"}]},\"type\":\"ConnectorPlacement.EquallySpacedConnector\",\"uuid\":\"ef76f81b-f821-49f2-9550-8127a934c8c3\"}],\"packageUris\":[\"http://schema.mathworks.com/mf0/Connector/R2020b\"],\"version\":\"1.0\"}"
  dq0 to abc : spsdq0toabcLib/dq0 to abc  Alignment=90 degrees behind phase A axis
  Va : PMIOPort  Side=Right
  Vb : PMIOPort  Port=2  Side=Right
  Vc : PMIOPort  Port=3  Side=Right
  Vabc : Outport
  Iabc : Outport  Port=2
  wires:
  Constant2/1 -> Voltage controller/2(Voq_ref)
  dq0 to abc/1 -> PWM Generator (2-Level)/1
  Subsystem/5(Ifd) -> Current controller/5(Ifd)
  Subsystem/2(Voq) -> Current controller/4(Voq), Voltage controller/4(Voq)
  Vod2_ref/1 -> Voltage controller/1(Vod_ref)
  Subsystem/6(Ifq) -> Current controller/6(Ifq)
  Subsystem/3(Iod) -> Voltage controller/5(iod)
  Voltage controller/2(ifq_ref) -> Current controller/2(Ifq_ref)
  Subsystem/4(Ioq) -> Voltage controller/6(ioq)
  Three-Phase V-I Measurement/2 -> Iabc/1, Subsystem/2(Io_abc)
  PWM Generator (2-Level)/1 -> Universal Bridge/1
  Constant/1 -> Mux/3
  Voltage controller/1(ifd_ref) -> Manual Switch1/1
  Current controller/2(mq) -> Mux/2
  Current controller/1(md) -> Mux/1
  Subsystem/1(Vod) -> Current controller/3(Vod), Voltage controller/3(Vod)
  Subsystem/7(wt) -> dq0 to abc/2
  Mux/1 -> dq0 to abc/1
  Three-Phase V-I Measurement/1 -> Scope/1, Subsystem/3(V0_abc), Vabc/1
  W/1 -> Subsystem/1(W), Current controller/7(W), Voltage controller/7(W)
  Three-Phase V-I Measurement1/2 -> Manual Switch/1
  Manual Switch/1 -> Subsystem/4(If_abc)
  Constant1/1 -> Manual Switch/2
  Constant3/1 -> Manual Switch1/2
  Manual Switch1/1 -> Current controller/1(Ifd_ref)
  connections:
  DC Voltage Source/LConn1 -- Universal Bridge/RConn2
  Three-Phase Series RLC Branch/LConn3 -- Three-Phase V-I Measurement1/RConn3
  Three-Phase Series RLC Branch/LConn1 -- Three-Phase V-I Measurement1/RConn1
  Three-Phase V-I Measurement/LConn1 -- Three-Phase Series RLC Branch2/LConn1 -- Three-Phase Series RLC Branch/RConn1
  Three-Phase V-I Measurement1/LConn1 -- Universal Bridge/LConn1
  Three-Phase Series RLC Branch/LConn2 -- Three-Phase V-I Measurement1/RConn2
  Three-Phase V-I Measurement/RConn1 -- Three-Phase Series RLC Branch1/LConn1
  Three-Phase V-I Measurement/RConn2 -- Three-Phase Series RLC Branch1/LConn2
  Three-Phase Series RLC Branch2/RConn1 -- Three-Phase Series RLC Branch2/RConn2 -- Three-Phase Series RLC Branch2/RConn3 -- Ground/LConn1
  DC Voltage Source/RConn1 -- Universal Bridge/RConn1
  Three-Phase V-I Measurement/LConn2 -- Three-Phase Series RLC Branch/RConn2 -- Three-Phase Series RLC Branch2/LConn2
  Three-Phase V-I Measurement/LConn3 -- Three-Phase Series RLC Branch/RConn3 -- Three-Phase Series RLC Branch2/LConn3
  Three-Phase V-I Measurement1/LConn2 -- Universal Bridge/LConn2
  Three-Phase V-I Measurement1/LConn3 -- Universal Bridge/LConn3
  Three-Phase V-I Measurement/RConn3 -- Three-Phase Series RLC Branch1/LConn3
  Vb/RConn1 -- Three-Phase Series RLC Branch1/RConn2
  Three-Phase Series RLC Branch1/RConn3 -- Vc/RConn1
  Three-Phase Series RLC Branch1/RConn1 -- Va/RConn1

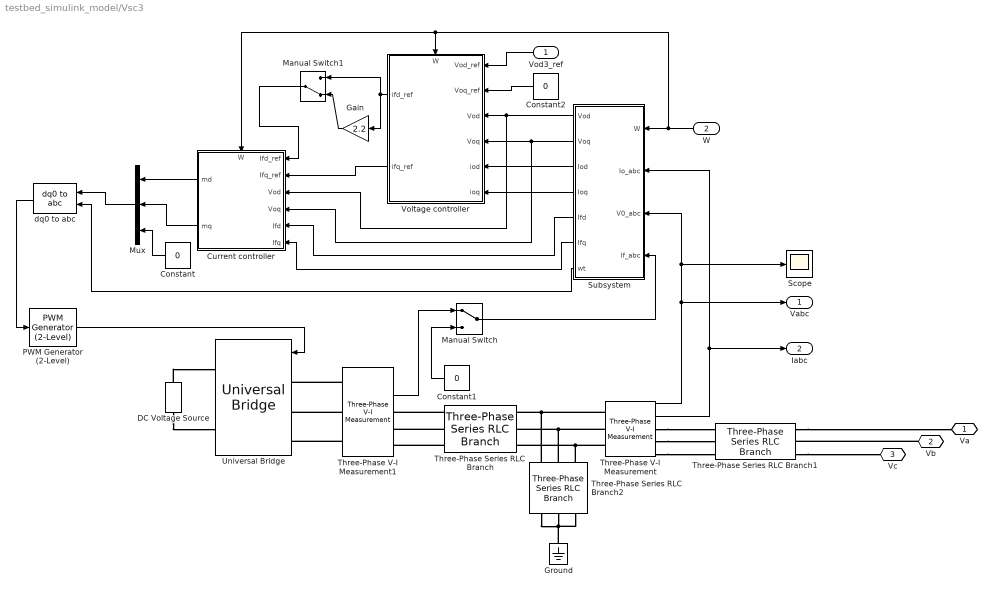
== system testbed_simulink_model/Vsc3 ==
  Vod3_ref : Inport
  W : Inport  Port=2
  Constant : Constant  Value=0
  Constant1 : Constant  Value=0
  Constant2 : Constant  Value=0
  Current controller : Subsystem
      settings: PortSchema="{\"entries\":[{\"content\":{\"sides\":[{\"content\":{\"connectorIds\":[\"In1\",\"In2\",\"In3\",\"In4\",\"In5\",\"In6\"]},\"type\":\"ConnectorPlacement.EquallySpacedRectSide\",\"uuid\":\"afbd0cd8-be12-4bd7-a6dd-f7dac5cf4512\"},{\"content\":{\"connectorIds\":[\"Out1\",\"Out2\"],\"side\":\"RIGHT\"},\"type\":\"ConnectorPlacement.EquallySpacedRectSide\",\"uuid\":\"a2288591-3041-41c1-b291-e9e060e5938f\"},{\"content\":{\"connectorIds\":[\"In7\"],\"side\":\"TOP\"},\"type\":\"ConnectorPlacement.EquallySpacedRectSide\",\"uuid\":\"6bd258a4-7022-4004-b2e3-8400b1f87dc6\"}]},\"type\":\"ConnectorPlacement.EquallySpacedConnector\",\"uuid\":\"ef76f81b-f821-49f2-9550-8127a934c8c3\"}],\"packageUris\":[\"http://schema.mathworks.com/mf0/Connector/R2020b\"],\"version\":\"1.0\"}"
  DC Voltage Source : spsDCVoltageSourceLib/DC Voltage Source  Amplitude=Vdc  Measurements=None
  Gain : Gain  Gain=2.2
  Ground : spsGroundLib/Ground  LConnTagsString=a
  Manual Switch : ManualSwitch
  Manual Switch1 : ManualSwitch  CurrentSetting=0
  Mux : Mux  Inputs=3
  PWM Generator (2-Level) : spsPWMGenerator2LevelLib/PWM Generator (2-Level)  ModulatorType=Three-phase bridge (6 pulses)  ModulatorMode=Unsynchronized  Fc=fsw  Pc=0  nF=27  MinMax="[ -1  1 ]"  SamplingTechnique=Natural  ModulatingSignals=off  m=0.8  Freq=60  Phase=0  Ts=0  ShowCarrierOutport=off
  Scope : Scope
  Subsystem : Subsystem
  Three-Phase Series RLC Branch : spsThreePhaseSeriesRLCBranchLib/Three-Phase Series RLC Branch  LConnTagsString=A|B|C  RConnTagsString=A|B|C  BranchType=RL  Resistance=Rf  Inductance=Lf  Capacitance=1e-6  Measurements=None
  Three-Phase Series RLC Branch1 : spsThreePhaseSeriesRLCBranchLib/Three-Phase Series RLC Branch  LConnTagsString=A|B|C  RConnTagsString=A|B|C  BranchType=RL  Resistance=Rc  Inductance=Lc  Capacitance=1e-6  Measurements=None
  Three-Phase Series RLC Branch2 : spsThreePhaseSeriesRLCBranchLib/Three-Phase Series RLC Branch  LConnTagsString=A|B|C  RConnTagsString=A|B|C  BranchType=C  Resistance=1  Inductance=1e-3  Capacitance=Cf  Measurements=None
  Three-Phase V-I Measurement : spsThreePhaseVIMeasurementLib/Three-Phase V-I Measurement  VoltageMeasurement=phase-to-ground  SetLabelV=off  LabelV=Vabc  Vpu=off  VpuLL=off  CurrentMeasurement=yes  SetLabelI=off  LabelI=Iabc  Ipu=off  Pbase=100e6  Vbase=500e3  OutputType=Complex  PhasorSimulation=off  PSBequivalent=0
  Three-Phase V-I Measurement1 : spsThreePhaseVIMeasurementLib/Three-Phase V-I Measurement  VoltageMeasurement=phase-to-ground  SetLabelV=off  LabelV=Vabc  Vpu=off  VpuLL=off  CurrentMeasurement=yes  SetLabelI=off  LabelI=Iabc  Ipu=off  Pbase=100e6  Vbase=500e3  OutputType=Complex  PhasorSimulation=off  PSBequivalent=0
  Universal Bridge : spsUniversalBridgeLib/Universal Bridge  Arms=3  SnubberResistance=1e5  SnubberCapacitance=inf  Device=IGBT / Diodes  Ron=1e-3  Lon=0  ForwardVoltages="[  0  0  ]"  ForwardVoltage=0  GTOparameters=[ 10e-6 , 20e-6 ]  IGBTparameters=[ 1e-6 , 2e-6 ]  Measurements=None  Measurements_2=None  converterType=Rectifier
  Voltage controller : Subsystem
      settings: PortSchema="{\"entries\":[{\"content\":{\"sides\":[{\"content\":{\"connectorIds\":[\"In1\",\"In2\",\"In3\",\"In4\",\"In5\",\"In6\"]},\"type\":\"ConnectorPlacement.EquallySpacedRectSide\",\"uuid\":\"afbd0cd8-be12-4bd7-a6dd-f7dac5cf4512\"},{\"content\":{\"connectorIds\":[\"Out1\",\"Out2\"],\"side\":\"RIGHT\"},\"type\":\"ConnectorPlacement.EquallySpacedRectSide\",\"uuid\":\"a2288591-3041-41c1-b291-e9e060e5938f\"},{\"content\":{\"connectorIds\":[\"In7\"],\"side\":\"TOP\"},\"type\":\"ConnectorPlacement.EquallySpacedRectSide\",\"uuid\":\"6bd258a4-7022-4004-b2e3-8400b1f87dc6\"}]},\"type\":\"ConnectorPlacement.EquallySpacedConnector\",\"uuid\":\"ef76f81b-f821-49f2-9550-8127a934c8c3\"}],\"packageUris\":[\"http://schema.mathworks.com/mf0/Connector/R2020b\"],\"version\":\"1.0\"}"
  dq0 to abc : spsdq0toabcLib/dq0 to abc  Alignment=90 degrees behind phase A axis
  Va : PMIOPort  Side=Right
  Vb : PMIOPort  Port=2  Side=Right
  Vc : PMIOPort  Port=3  Side=Right
  Vabc : Outport
  Iabc : Outport  Port=2
  wires:
  Constant2/1 -> Voltage controller/2(Voq_ref)
  dq0 to abc/1 -> PWM Generator (2-Level)/1
  Subsystem/5(Ifd) -> Current controller/5(Ifd)
  Subsystem/2(Voq) -> Current controller/4(Voq), Voltage controller/4(Voq)
  Vod3_ref/1 -> Voltage controller/1(Vod_ref)
  Subsystem/6(Ifq) -> Current controller/6(Ifq)
  Subsystem/3(Iod) -> Voltage controller/5(iod)
  Voltage controller/2(ifq_ref) -> Current controller/2(Ifq_ref)
  Subsystem/4(Ioq) -> Voltage controller/6(ioq)
  Three-Phase V-I Measurement/2 -> Iabc/1, Subsystem/2(Io_abc)
  PWM Generator (2-Level)/1 -> Universal Bridge/1
  Constant/1 -> Mux/3
  Voltage controller/1(ifd_ref) -> Gain/1, Manual Switch1/1
  Current controller/2(mq) -> Mux/2
  Current controller/1(md) -> Mux/1
  Subsystem/1(Vod) -> Current controller/3(Vod), Voltage controller/3(Vod)
  Subsystem/7(wt) -> dq0 to abc/2
  Mux/1 -> dq0 to abc/1
  Three-Phase V-I Measurement/1 -> Vabc/1, Scope/1, Subsystem/3(V0_abc)
  W/1 -> Subsystem/1(W), Current controller/7(W), Voltage controller/7(W)
  Constant1/1 -> Manual Switch/2
  Three-Phase V-I Measurement1/2 -> Manual Switch/1
  Manual Switch/1 -> Subsystem/4(If_abc)
  Gain/1 -> Manual Switch1/2
  Manual Switch1/1 -> Current controller/1(Ifd_ref)
  connections:
  DC Voltage Source/LConn1 -- Universal Bridge/RConn2
  Three-Phase Series RLC Branch/LConn3 -- Three-Phase V-I Measurement1/RConn3
  Three-Phase Series RLC Branch/LConn1 -- Three-Phase V-I Measurement1/RConn1
  Three-Phase V-I Measurement/LConn1 -- Three-Phase Series RLC Branch2/LConn1 -- Three-Phase Series RLC Branch/RConn1
  Three-Phase V-I Measurement1/LConn1 -- Universal Bridge/LConn1
  Three-Phase Series RLC Branch/LConn2 -- Three-Phase V-I Measurement1/RConn2
  Three-Phase V-I Measurement/RConn1 -- Three-Phase Series RLC Branch1/LConn1
  Three-Phase V-I Measurement/RConn2 -- Three-Phase Series RLC Branch1/LConn2
  Three-Phase Series RLC Branch2/RConn1 -- Three-Phase Series RLC Branch2/RConn2 -- Three-Phase Series RLC Branch2/RConn3 -- Ground/LConn1
  DC Voltage Source/RConn1 -- Universal Bridge/RConn1
  Three-Phase V-I Measurement/LConn2 -- Three-Phase Series RLC Branch2/LConn2 -- Three-Phase Series RLC Branch/RConn2
  Three-Phase V-I Measurement/LConn3 -- Three-Phase Series RLC Branch2/LConn3 -- Three-Phase Series RLC Branch/RConn3
  Three-Phase V-I Measurement1/LConn2 -- Universal Bridge/LConn2
  Three-Phase V-I Measurement1/LConn3 -- Universal Bridge/LConn3
  Three-Phase V-I Measurement/RConn3 -- Three-Phase Series RLC Branch1/LConn3
  Vb/RConn1 -- Three-Phase Series RLC Branch1/RConn2
  Three-Phase Series RLC Branch1/RConn3 -- Vc/RConn1
  Three-Phase Series RLC Branch1/RConn1 -- Va/RConn1

== system testbed_simulink_model/Droop control1/Subsystem ==
  V0_abc : Inport
  Io_abc : Inport  Port=2
  W : Inport  Port=3
  Demux : Demux  Outputs=3
  Demux2 : Demux  Outputs=3
  Integrator : Integrator
  Terminator : Terminator
  Terminator2 : Terminator
  abc to dq0 : spsabctodq0Lib/abc to dq0  Alignment=90 degrees behind phase A axis
  abc to dq2 : spsabctodq0Lib/abc to dq0  Alignment=90 degrees behind phase A axis
  wt : Outport
  Vod : Outport  Port=2
  Voq : Outport  Port=3
  Iod : Outport  Port=4
  Ioq : Outport  Port=5
  wires:
  abc to dq2/1 -> Demux2/1
  Demux/2 -> Voq/1
  Integrator/1 -> wt/1, abc to dq2/2, abc to dq0/2
  Demux2/2 -> Ioq/1
  abc to dq0/1 -> Demux/1
  Demux2/3 -> Terminator2/1
  Demux2/1 -> Iod/1
  Demux/1 -> Vod/1
  Demux/3 -> Terminator/1
  W/1 -> Integrator/1
  Io_abc/1 -> abc to dq2/1
  V0_abc/1 -> abc to dq0/1

== system testbed_simulink_model/Droop control2/Subsystem ==
  V0_abc : Inport
  Io_abc : Inport  Port=2
  W : Inport  Port=3
  Demux : Demux  Outputs=3
  Demux2 : Demux  Outputs=3
  Integrator : Integrator
  Terminator : Terminator
  Terminator2 : Terminator
  abc to dq0 : spsabctodq0Lib/abc to dq0  Alignment=90 degrees behind phase A axis
  abc to dq2 : spsabctodq0Lib/abc to dq0  Alignment=90 degrees behind phase A axis
  wt : Outport
  Vod : Outport  Port=2
  Voq : Outport  Port=3
  Iod : Outport  Port=4
  Ioq : Outport  Port=5
  wires:
  abc to dq2/1 -> Demux2/1
  Demux/2 -> Voq/1
  Integrator/1 -> wt/1, abc to dq2/2, abc to dq0/2
  Demux2/2 -> Ioq/1
  abc to dq0/1 -> Demux/1
  Demux2/3 -> Terminator2/1
  Demux2/1 -> Iod/1
  Demux/1 -> Vod/1
  Demux/3 -> Terminator/1
  W/1 -> Integrator/1
  Io_abc/1 -> abc to dq2/1
  V0_abc/1 -> abc to dq0/1

== system testbed_simulink_model/Droop control3/Subsystem ==
  V0_abc : Inport
  Io_abc : Inport  Port=2
  W : Inport  Port=3
  Demux : Demux  Outputs=3
  Demux2 : Demux  Outputs=3
  Integrator : Integrator
  Terminator : Terminator
  Terminator2 : Terminator
  abc to dq0 : spsabctodq0Lib/abc to dq0  Alignment=90 degrees behind phase A axis
  abc to dq2 : spsabctodq0Lib/abc to dq0  Alignment=90 degrees behind phase A axis
  wt : Outport
  Vod : Outport  Port=2
  Voq : Outport  Port=3
  Iod : Outport  Port=4
  Ioq : Outport  Port=5
  wires:
  abc to dq2/1 -> Demux2/1
  Demux/2 -> Voq/1
  Integrator/1 -> wt/1, abc to dq2/2, abc to dq0/2
  Demux2/2 -> Ioq/1
  abc to dq0/1 -> Demux/1
  Demux2/3 -> Terminator2/1
  Demux2/1 -> Iod/1
  Demux/1 -> Vod/1
  Demux/3 -> Terminator/1
  W/1 -> Integrator/1
  Io_abc/1 -> abc to dq2/1
  V0_abc/1 -> abc to dq0/1

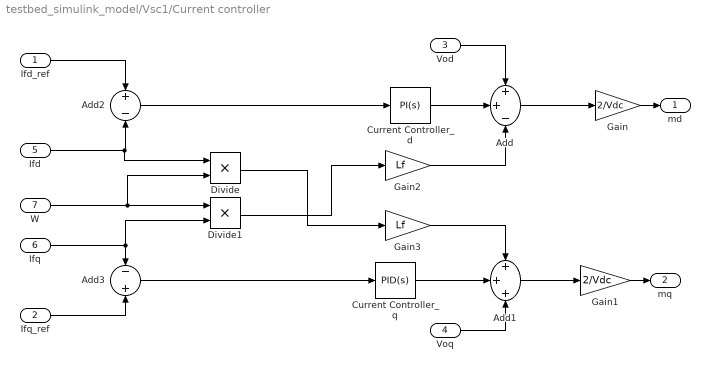
== system testbed_simulink_model/Vsc1/Current controller ==
  Ifd_ref : Inport
  Ifq_ref : Inport  Port=2
  Vod : Inport  Port=3
  Voq : Inport  Port=4
  Ifd : Inport  Port=5
  Ifq : Inport  Port=6
  W : Inport  Port=7
  Add : Sum  Inputs=++-
  Add1 : Sum  Inputs=+++
  Add2 : Sum  Inputs=+-
  Add3 : Sum  Inputs=-+
  Current Controller_d : pid_lib/PID Controller  Controller=PI  Form=Parallel  TimeDomain=Continuous-time  UseExternalTs=off  SampleTime=-1  IntegratorMethod=Forward Euler  FilterMethod=Forward Euler  ControllerParametersSource=internal  P=Kpc  I=Kic  D=0  UseFilter=on  N=100  TunerSelectOption=Transfer Function Based (PID Tuner App)  InitialConditionSource=internal  InitialConditionForIntegrator=0  InitialConditionForFilter=0  DifferentiatorICPrevScaledInput=0  ExternalReset=none  TrackingMode=off  Kt=1  LimitOutput=off  SatLimitsSource=internal  UpperSaturationLimit=inf  LowerSaturationLimit=-inf  LinearizeAsGain=on  AntiWindupMode=none  Kb=1  POutMin=[]  POutMax=[]  IOutMin=[]  IOutMax=[]  DOutMin=[]  DOutMax=[]  NOutMin=[]  NOutMax=[]  SumOutMin=[]  SumOutMax=[]  SaturationOutMin=[]  SaturationOutMax=[]  PParamMin=[]  PParamMax=[]  IParamMin=[]  IParamMax=[]  DParamMin=[]  DParamMax=[]  NParamMin=[]  NParamMax=[]  KbParamMin=[]  KbParamMax=[]  KtParamMin=[]  KtParamMax=[]  KbOutMin=[]  KbOutMax=[]  KtOutMin=[]  KtOutMax=[]  IntegratorOutMin=[]  IntegratorOutMax=[]  FilterOutMin=[]  FilterOutMax=[]  SumI1OutMin=[]  SumI1OutMax=[]  SumI2OutMin=[]  SumI2OutMax=[]  SumI3OutMin=[]  SumI3OutMax=[]  SumI4OutMin=[]  SumI4OutMax=[]  SumDOutMin=[]  SumDOutMax=[]  DifferentiatorOutMin=[]  DifferentiatorOutMax=[]  FilterDiffOutCoefMin=[]  FilterDiffOutCoefMax=[]  ReciprocalOutMin=[]  ReciprocalOutMax=[]  SumDenOutMin=[]  SumDenOutMax=[]  SumNumOutMin=[]  SumNumOutMax=[]  DivideOutMin=[]  DivideOutMax=[]  UdiffTsProdOutMin=[]  UdiffTsProdOutMax=[]  NTsProdOutMin=[]  NTsProdOutMax=[]  UintegralTsProdOutMin=[]  UintegralTsProdOutMax=[]  UngainTsProdOutMin=[]  UngainTsProdOutMax=[]  IntegratorContinuousStateAttributes=''  IntegratorStateMustResolveToSignalObject=off  IntegratorRTWStateStorageClass=Auto  FilterContinuousStateAttributes=''  FilterStateMustResolveToSignalObject=off  FilterRTWStateStorageClass=Auto  ParallelPVariant=InternalParameters  IdealPVariant=Disabled  IVariant=InternalParameters  DVariant=Disabled  IntegratorVariant=Continuous  SatVariant=Disabled  AWVariant=Passthrough  PCopyVariant=Disabled  TRVariant=Disabled  FdbkBlocksVariant=Forward  IdealPFdbkVariant=Disabled  SatFdbkVariant=Disabled  DerivativeFilterVariant=Disabled  NVariant=Disabled  NCopyVariant=Disabled_SignalSpec  FilterICVariant=Disabled  IntegratorICVariant=InternalICs  ExternalResetVariant=Disabled  TRSumVariant=Passthrough  SumFdbkVariant=Disabled  SumVariant=Sum_PI  TsampFilterVariant=InternalTs  TsampNgainVariant=Passthrough  TsampIntegralVariant=Passthrough  ExternalSaturationOutDataTypeStr=Inherit: Same as second input
  Current Controller_q : pid_lib/PID Controller  Controller=PID  Form=Parallel  TimeDomain=Continuous-time  UseExternalTs=off  SampleTime=-1  IntegratorMethod=Forward Euler  FilterMethod=Forward Euler  ControllerParametersSource=internal  P=Kpc  I=Kic  D=0  UseFilter=on  N=100  TunerSelectOption=Transfer Function Based (PID Tuner App)  InitialConditionSource=internal  InitialConditionForIntegrator=0  InitialConditionForFilter=0  DifferentiatorICPrevScaledInput=0  ExternalReset=none  TrackingMode=off  Kt=1  LimitOutput=off  SatLimitsSource=internal  UpperSaturationLimit=inf  LowerSaturationLimit=-inf  LinearizeAsGain=on  AntiWindupMode=none  Kb=1  POutMin=[]  POutMax=[]  IOutMin=[]  IOutMax=[]  DOutMin=[]  DOutMax=[]  NOutMin=[]  NOutMax=[]  SumOutMin=[]  SumOutMax=[]  SaturationOutMin=[]  SaturationOutMax=[]  PParamMin=[]  PParamMax=[]  IParamMin=[]  IParamMax=[]  DParamMin=[]  DParamMax=[]  NParamMin=[]  NParamMax=[]  KbParamMin=[]  KbParamMax=[]  KtParamMin=[]  KtParamMax=[]  KbOutMin=[]  KbOutMax=[]  KtOutMin=[]  KtOutMax=[]  IntegratorOutMin=[]  IntegratorOutMax=[]  FilterOutMin=[]  FilterOutMax=[]  SumI1OutMin=[]  SumI1OutMax=[]  SumI2OutMin=[]  SumI2OutMax=[]  SumI3OutMin=[]  SumI3OutMax=[]  SumI4OutMin=[]  SumI4OutMax=[]  SumDOutMin=[]  SumDOutMax=[]  DifferentiatorOutMin=[]  DifferentiatorOutMax=[]  FilterDiffOutCoefMin=[]  FilterDiffOutCoefMax=[]  ReciprocalOutMin=[]  ReciprocalOutMax=[]  SumDenOutMin=[]  SumDenOutMax=[]  SumNumOutMin=[]  SumNumOutMax=[]  DivideOutMin=[]  DivideOutMax=[]  UdiffTsProdOutMin=[]  UdiffTsProdOutMax=[]  NTsProdOutMin=[]  NTsProdOutMax=[]  UintegralTsProdOutMin=[]  UintegralTsProdOutMax=[]  UngainTsProdOutMin=[]  UngainTsProdOutMax=[]  IntegratorContinuousStateAttributes=''  IntegratorStateMustResolveToSignalObject=off  IntegratorRTWStateStorageClass=Auto  FilterContinuousStateAttributes=''  FilterStateMustResolveToSignalObject=off  FilterRTWStateStorageClass=Auto  ParallelPVariant=InternalParameters  IdealPVariant=Disabled  IVariant=InternalParameters  DVariant=InternalParameters  IntegratorVariant=Continuous  SatVariant=Disabled  AWVariant=Passthrough  PCopyVariant=Disabled  TRVariant=Disabled  FdbkBlocksVariant=Forward  IdealPFdbkVariant=Disabled  SatFdbkVariant=Disabled  DerivativeFilterVariant=ContFilter  NVariant=InternalParameters  NCopyVariant=Disabled  FilterICVariant=InternalICsFilter  IntegratorICVariant=InternalICs  ExternalResetVariant=Disabled  TRSumVariant=Passthrough  SumFdbkVariant=Disabled  SumVariant=Sum_PID  TsampFilterVariant=InternalTs  TsampNgainVariant=Passthrough  TsampIntegralVariant=Passthrough  ExternalSaturationOutDataTypeStr=Inherit: Same as second input
  Divide : Product  Inputs=**
  Divide1 : Product  Inputs=**
  Gain : Gain  Gain=2/Vdc
  Gain1 : Gain  Gain=2/Vdc
  Gain2 : Gain  Gain=Lf
  Gain3 : Gain  Gain=Lf
  md : Outport
  mq : Outport  Port=2
  wires:
  Voq/1 -> Add1/3
  Ifd_ref/1 -> Add2/1
  Ifq_ref/1 -> Add3/2
  Gain3/1 -> Add1/1
  Current Controller_q/1 -> Add1/2
  Gain2/1 -> Add/3
  Vod/1 -> Add/1
  Add/1 -> Gain/1
  Add2/1 -> Current Controller_d/1
  Add3/1 -> Current Controller_q/1
  Add1/1 -> Gain1/1
  Current Controller_d/1 -> Add/2
  Gain1/1 -> mq/1
  Gain/1 -> md/1
  Ifd/1 -> Divide/1, Add2/2
  Divide/1 -> Gain3/1
  W/1 -> Divide1/1, Divide/2
  Divide1/1 -> Gain2/1
  Ifq/1 -> Add3/1, Divide1/2

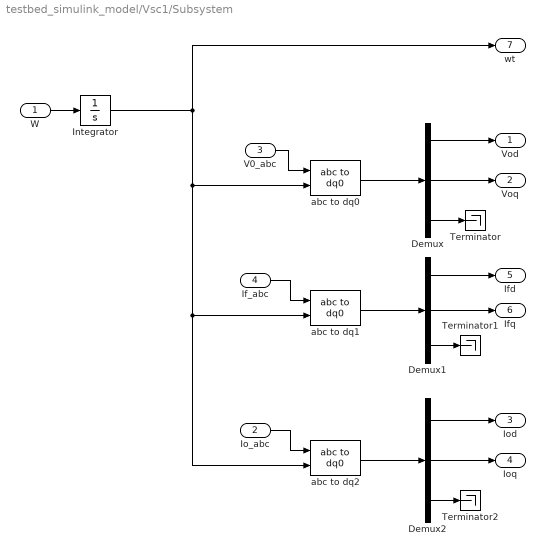
== system testbed_simulink_model/Vsc1/Subsystem ==
  W : Inport
  Io_abc : Inport  Port=2
  V0_abc : Inport  Port=3
  If_abc : Inport  Port=4
  Demux : Demux  Outputs=3
  Demux1 : Demux  Outputs=3
  Demux2 : Demux  Outputs=3
  Integrator : Integrator
  Terminator : Terminator
  Terminator1 : Terminator
  Terminator2 : Terminator
  abc to dq0 : spsabctodq0Lib/abc to dq0  Alignment=90 degrees behind phase A axis
  abc to dq1 : spsabctodq0Lib/abc to dq0  Alignment=90 degrees behind phase A axis
  abc to dq2 : spsabctodq0Lib/abc to dq0  Alignment=90 degrees behind phase A axis
  Vod : Outport
  Voq : Outport  Port=2
  Iod : Outport  Port=3
  Ioq : Outport  Port=4
  Ifd : Outport  Port=5
  Ifq : Outport  Port=6
  wt : Outport  Port=7
  wires:
  Demux2/3 -> Terminator2/1
  Demux/3 -> Terminator/1
  abc to dq0/1 -> Demux/1
  Demux2/2 -> Ioq/1
  Demux2/1 -> Iod/1
  abc to dq1/1 -> Demux1/1
  Demux1/2 -> Ifq/1
  Demux1/1 -> Ifd/1
  abc to dq2/1 -> Demux2/1
  Demux1/3 -> Terminator1/1
  If_abc/1 -> abc to dq1/1
  Integrator/1 -> abc to dq2/2, abc to dq1/2, abc to dq0/2, wt/1
  V0_abc/1 -> abc to dq0/1
  Io_abc/1 -> abc to dq2/1
  W/1 -> Integrator/1
  Demux/2 -> Voq/1
  Demux/1 -> Vod/1
